simulink model "Testbench_EthernetCommunication"  (R2019b)
settings: Solver=ode1  StartTime=0.0  StopTime=Inf  RelTol=1e-3
PostLoadFcn:
  | , if any(exist('dsrtsu_mdlpostloadfcn', 'file') == [2, 3, 6]), try dsrtsu_mdlpostloadfcn('Execute', bdroot); catch fprintf('Error in PostLoadFcn (dsrtsu_mdlpostloadfcn) for model "%s":\n %s\n', bdroot, lasterr); end, end,
libraries: Lib_EthernetCommunication x1
settings Model: DSRTSU_INTERNAL_RTI_VER=550  DSRTSU_INTERNAL_RTI_TYPE=rti1401  RTICANMMDATA=struct('GeneralSetupData',struct('modelroot','C:\Users\kessler\Documents\fav\apollo_opensource\modules\autobox_control\libraries','generalsettings',struct('filesettings',struct('destfolder',struct('Name','RTICANMM_FILES','Check',1),'buildfolder',struct('Name','.','Check',1),'AbsDestfolder',struct('Name','C:\Users\kessler\Documents\fav\apollo_opensource\modules\autobox_control\libraries\RTICANMM_FILES'),'AbsBuildfolder',struct('Name','C:\Users\kessler\Documents\fav\apollo_opensource\modules\autobox_control\libraries'))),'options',struct('addpaths',1,'rmpaths',1,'addtrcexclusion',true,'cannavigator',struct('checkmonitoring',0),'show_usrtrc',0,'use_usrtrc',0),'advanced',struct('options',ones(1,100)),'MPSetup',{{}},'RTI',struct('Type','GRT','Ver','','Date',''),'modelname','Testbench_EthernetCommunication','block','Testbench_EthernetCommunication'))  DSRTSU_INTERNAL_RTIFPGA=150  Creator=esterle  LastModifiedBy=kessler
settings DataIOCC: ReturnWorkspaceOutputs=off
settings DebuggingCC: ArithmeticOperatorsInVariantConditions=warning
settings SFSimCC: SimUseLocalCustomCode=off  CustomCodeUndefinedFunction=UseInterfaceOnly
settings RTWCC: RTWUseLocalCustomCode=off

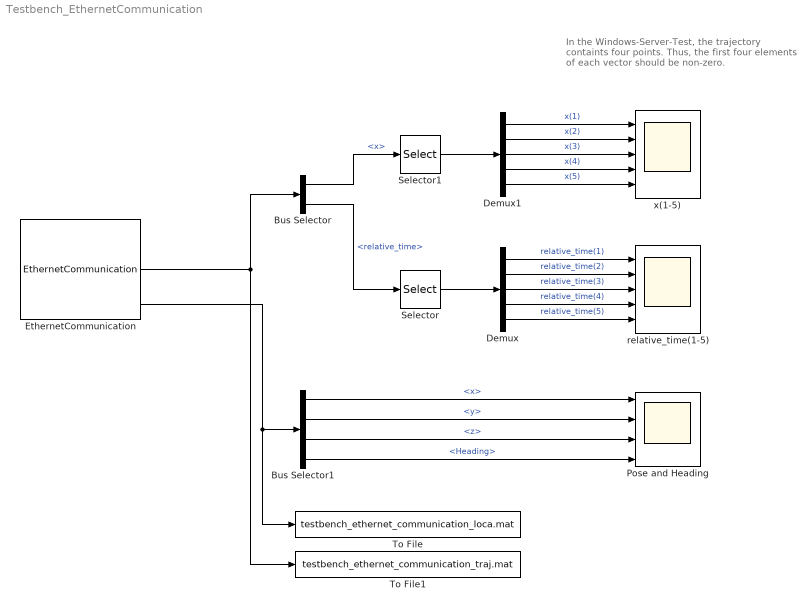
== system Testbench_EthernetCommunication ==
  note: In the Windows-Server-Test, the trajectory containts four points. Thus, the first four elements of each vector should be non-zero.
  Bus Selector : BusSelector  OutputSignals=x,relative_time
  Bus Selector1 : BusSelector  OutputSignals=Pose.Position.x,Pose.Position.y,Pose.Position.z,Pose.Heading
  Demux : Demux  Outputs=5
  Demux1 : Demux  Outputs=5
  EthernetCommunication : Lib_EthernetCommunication/EthernetCommunication  SystemSampleTime=-1  Latency=0  AutoFrameSizeCalculation=off
  Pose and Heading : Scope  NumInputPorts=4
  Selector : Selector  InputPortWidth=1000  IndexOptions=Index vector (dialog)  Indices=[1 2 3 4 5]  OutputSizes=1
  Selector1 : Selector  InputPortWidth=1000  IndexOptions=Index vector (dialog)  Indices=[1 2 3 4 5]  OutputSizes=1
  To File : ToFile  Filename=testbench_ethernet_communication_loca.mat  MatrixName=localization  SaveFormat=Timeseries
  To File1 : ToFile  Filename=testbench_ethernet_communication_traj.mat  MatrixName=trajectory  SaveFormat=Timeseries
  relative_time(1-5) : Scope  NumInputPorts=5
  x(1-5) : Scope  NumInputPorts=5
  wires:
  EthernetCommunication/2 -> To File1/1, Bus Selector/1
  Bus Selector/2 -> Selector/1  "<relative_time>"
  Selector/1 -> Demux/1
  Demux/1 -> relative_time(1-5)/1  "relative_time(1)"
  Demux/2 -> relative_time(1-5)/2  "relative_time(2)"
  Demux/3 -> relative_time(1-5)/3  "relative_time(3)"
  Demux/4 -> relative_time(1-5)/4  "relative_time(4)"
  Demux/5 -> relative_time(1-5)/5  "relative_time(5)"
  Demux1/2 -> x(1-5)/2  "x(2)"
  Demux1/3 -> x(1-5)/3  "x(3)"
  Demux1/1 -> x(1-5)/1  "x(1)"
  Selector1/1 -> Demux1/1
  Demux1/5 -> x(1-5)/5  "x(5)"
  Demux1/4 -> x(1-5)/4  "x(4)"
  Bus Selector/1 -> Selector1/1  "<x>"
  EthernetCommunication/3 -> To File/1, Bus Selector1/1
  Bus Selector1/1 -> Pose and Heading/1  "<x>"
  Bus Selector1/2 -> Pose and Heading/2  "<y>"
  Bus Selector1/3 -> Pose and Heading/3  "<z>"
  Bus Selector1/4 -> Pose and Heading/4  "<Heading>"
